simulink model "model_dyskretny_2"  (R2020a)
settings: Solver=VariableStepAuto  StartTime=0.0  StopTime=10.0  RelTol=1e-3
values from neighbouring files (symbols this model uses):
  ic = 0.0    (= 0)    [pom.m]    (also in zad1_4.m = 0.01)
  T = 0.5    [pom.m]    (also in zad1_10.m; zad1_4.m; zad1_6_1.m; zad1_6_2.m)
settings Model: Creator=jakub  LastModifiedBy=jakub

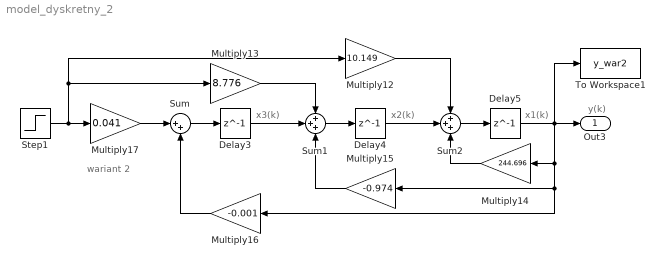
== system model_dyskretny_2 ==
  note: x1(k)
  note: wariant 2
  note: x2(k)
  note: y(k)
  note: x3(k)
  Delay3 : Delay  DelayLength=1  InitialCondition=ic  SampleTime=T
  Delay4 : Delay  DelayLength=1  InitialCondition=ic  SampleTime=T
  Delay5 : Delay  DelayLength=1  InitialCondition=ic  SampleTime=T
  Multiply12 : Gain  Gain=10.149
  Multiply13 : Gain  Gain=8.776
  Multiply14 : Gain  Gain=244.696
  Multiply15 : Gain  Gain=-0.974
  Multiply16 : Gain  Gain=-0.001
  Multiply17 : Gain  Gain=0.041
  Step1 : Step  SampleTime=0
  Sum : Sum  Inputs=|++
  Sum1 : Sum  Inputs=+++
  Sum2 : Sum  Inputs=+++
  To Workspace1 : ToWorkspace  VariableName=y_war2  SaveFormat=Structure With Time  SampleTime=T
  Out3 : Outport
  wires:
  Delay3/1 -> Sum1/2
  Multiply16/1 -> Sum/2
  Delay5/1 -> To Workspace1/1, Multiply16/1, Multiply15/1, Multiply14/1, Out3/1
  Multiply12/1 -> Sum2/1
  Multiply13/1 -> Sum1/1
  Multiply14/1 -> Sum2/3
  Sum2/1 -> Delay5/1
  Sum1/1 -> Delay4/1
  Multiply15/1 -> Sum1/3
  Delay4/1 -> Sum2/2
  Multiply17/1 -> Sum/1
  Step1/1 -> Multiply17/1, Multiply12/1, Multiply13/1
  Sum/1 -> Delay3/1
